simulink model "simulator"  (R2024a)
settings: Solver=VariableStepAuto  StartTime=0.0  StopTime=10  RelTol=1e-3
undefined symbols (not defined in the file): desiredState, params, x0
libraries: simulink x2, matrix_library x1
settings Model: Creator=matteocolussi  LastModifiedBy=matteocolussi

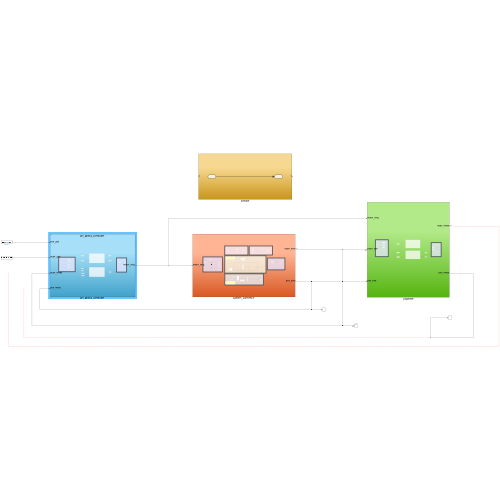
[thumbnail: Simulink's stored preview of the top-level diagram]
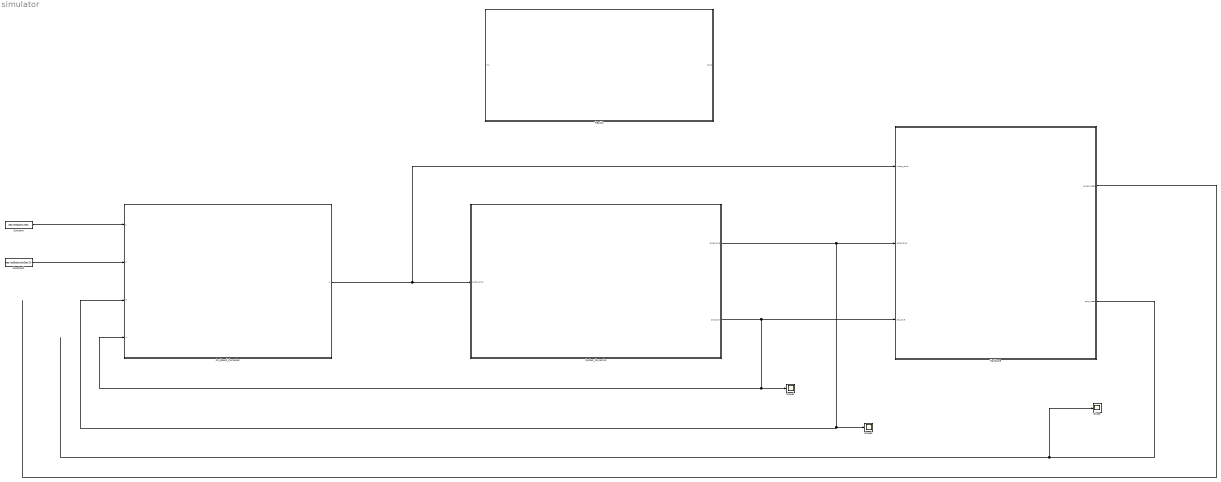
== system simulator ==
  Constant : Constant  Value=desiredState.rDes
  Constant1 : Constant  Value=desiredState.attDes(3)
  Hardware : Subsystem
  On_Board_Computer : Subsystem  ReferencedSubsystem=On_Board_Computer
  Results : Subsystem
  Scope : Scope
  Scope1 : Scope
  Scope2 : Scope
  System_Dynamics : Subsystem
  wires:
  On_Board_Computer/1 -> Hardware/1(motor_cmd), System_Dynamics/1(motor_cmd)
  System_Dynamics/1(euler_true) -> Hardware/2(euler_true), On_Board_Computer/3, Scope2/1
  System_Dynamics/2(pos_true) -> Scope1/1, On_Board_Computer/4, Hardware/3(pos_true)
  Hardware/1(euler_meas) -> ?
  Hardware/2(pos_meas) -> Scope/1
  Constant/1 -> On_Board_Computer/1
  Constant1/1 -> On_Board_Computer/2

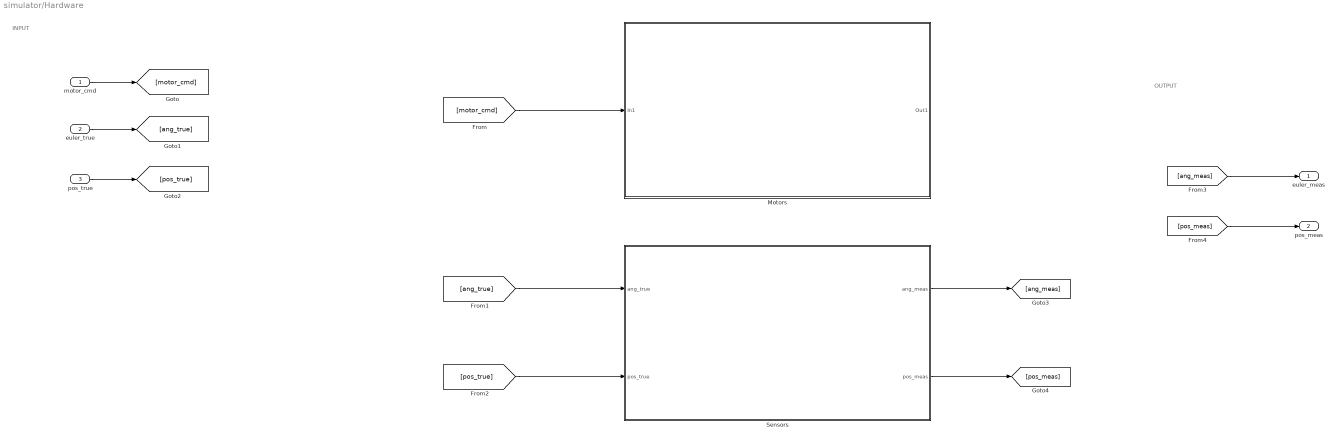
== system simulator/Hardware ==
  note: INPUT
  note: OUTPUT
  motor_cmd : Inport
  euler_true : Inport  Port=2
  pos_true : Inport  Port=3
  Motors : Subsystem
  Sensors : Subsystem
  euler_meas : Outport
  pos_meas : Outport  Port=2
  wires:
  motor_cmd/1 -> [motor_cmd]
  [motor_cmd] -> Motors/1(In1)
  euler_true/1 -> [ang_true]
  pos_true/1 -> [pos_true]
  [ang_true] -> Sensors/1(ang_true)
  [pos_true] -> Sensors/2(pos_true)
  Sensors/1(ang_meas) -> [ang_meas]
  Sensors/2(pos_meas) -> [pos_meas]
  [ang_meas] -> euler_meas/1
  [pos_meas] -> pos_meas/1

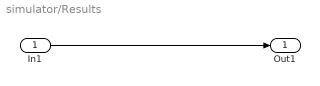
== system simulator/Results ==
  In1 : Inport
  Out1 : Outport
  wires:
  In1/1 -> Out1/1

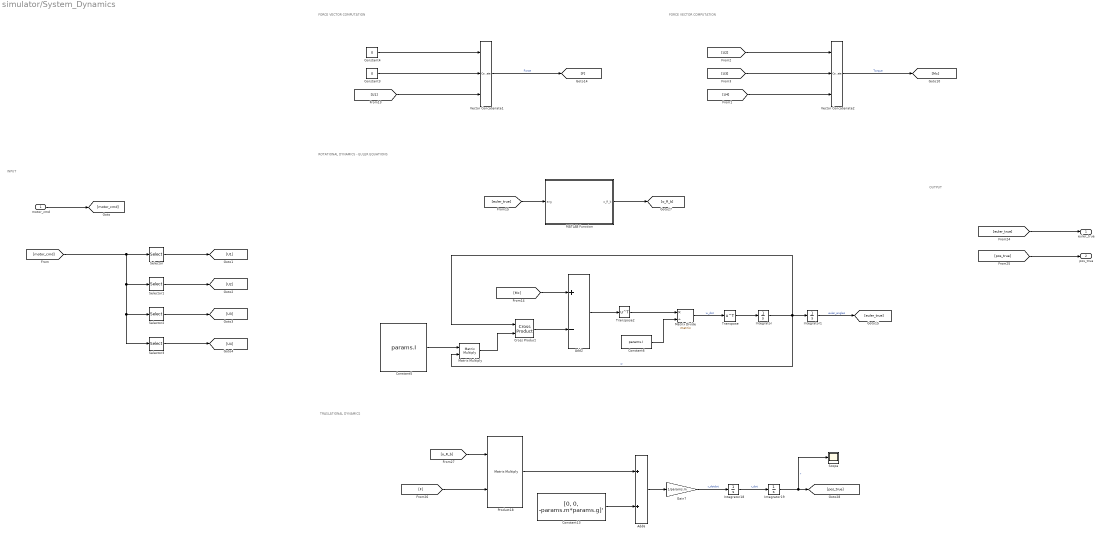
== system simulator/System_Dynamics ==
  note: ROTATIONAL DYNAMICS - EULER EQUATIONS
  note: FORCE VECTOR COMPUTATION
  note: INPUT
  note: OUTPUT
  note: TRASLATIONAL DYNAMICS
  note: FORCE VECTOR COMPUTATION
  motor_cmd : Inport
  Add2 : Sum  Inputs=+-
  Add6 : Sum
  Constant13 : Constant  Value=[0, 0, -params.m*params.g]'
  Constant3 : Constant  Value=0
  Constant4 : Constant  Value=0
  Constant5 : Constant  Value=params.I  VectorParams1D=off
  Constant6 : Constant  Value=params.I
  Cross Product : matrix_library/Cross Product
  Gain7 : Gain  Gain=1/params.m
  Integrator : Integrator
  Integrator1 : Integrator  InitialCondition=x0(7:9)
  Integrator18 : Integrator
  Integrator19 : Integrator  InitialCondition=x0(1:3);
  MATLAB Function : MATLAB Function  TreatAsAtomicUnit=on
  Matrix Divide : Product  Inputs=*/  Multiplication=Matrix(*)
  Matrix Multiply : Product  Multiplication=Matrix(*)
  Product18 : Product  Multiplication=Matrix(*)
  Scope : Scope
  Selector : Selector  InputPortWidth=4  IndexOptions=Index vector (dialog)  Indices=1  OutputSizes=1
  Selector1 : Selector  InputPortWidth=4  IndexOptions=Index vector (dialog)  Indices=2  OutputSizes=1
  Selector2 : Selector  InputPortWidth=4  IndexOptions=Index vector (dialog)  Indices=3  OutputSizes=1
  Selector3 : Selector  InputPortWidth=4  IndexOptions=Index vector (dialog)  Indices=4  OutputSizes=1
  Transpose : Math  Operator=transpose
  Transpose2 : Math  Operator=transpose
  Vector Concatenate1 : Concatenate  NumInputs=3
  Vector Concatenate2 : Concatenate  NumInputs=3
  euler_true : Outport
  pos_true : Outport  Port=2
  wires:
  motor_cmd/1 -> [motor_cmd]
  Selector/1 -> [U1]
  Selector1/1 -> [U2]
  Selector2/1 -> [U3]
  [motor_cmd] -> Selector3/1, Selector2/1, Selector1/1, Selector/1
  Selector3/1 -> [U4]
  [U1] -> Vector Concatenate1/3
  Constant3/1 -> Vector Concatenate1/2
  Constant4/1 -> Vector Concatenate1/1
  Vector Concatenate1/1 -> [F]  "Force"
  [euler_true] -> MATLAB Function/1(ang)
  MATLAB Function/1(o_R_b) -> [o_R_b]
  [euler_true] -> euler_true/1
  [pos_true] -> pos_true/1
  Add6/1 -> Gain7/1
  [F] -> Product18/2
  Product18/1 -> Add6/1
  Gain7/1 -> Integrator18/1  "r_dotdot"
  [o_R_b] -> Product18/1
  Constant13/1 -> Add6/2
  Integrator18/1 -> Integrator19/1  "r_dot"
  Integrator19/1 -> [pos_true], Scope/1  "r"
  Constant5/1 -> Matrix Multiply/1
  Matrix Multiply/1 -> Cross Product/2
  Cross Product/1 -> Add2/2
  Add2/1 -> Transpose2/1
  Constant6/1 -> Matrix Divide/2
  Matrix Divide/1 -> Transpose/1  "w_dot"
  Integrator/1 -> Integrator1/1, Cross Product/1, Matrix Multiply/2  "w"
  Integrator1/1 -> [euler_true]  "euler_angles"
  [U2] -> Vector Concatenate2/1
  Vector Concatenate2/1 -> [Mc]  "Torque"
  [U4] -> Vector Concatenate2/3
  [U3] -> Vector Concatenate2/2
  Transpose/1 -> Integrator/1
  [Mc] -> Add2/1
  Transpose2/1 -> Matrix Divide/1

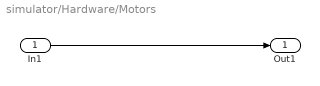
== system simulator/Hardware/Motors ==
  In1 : Inport
  Out1 : Outport
  wires:
  In1/1 -> Out1/1

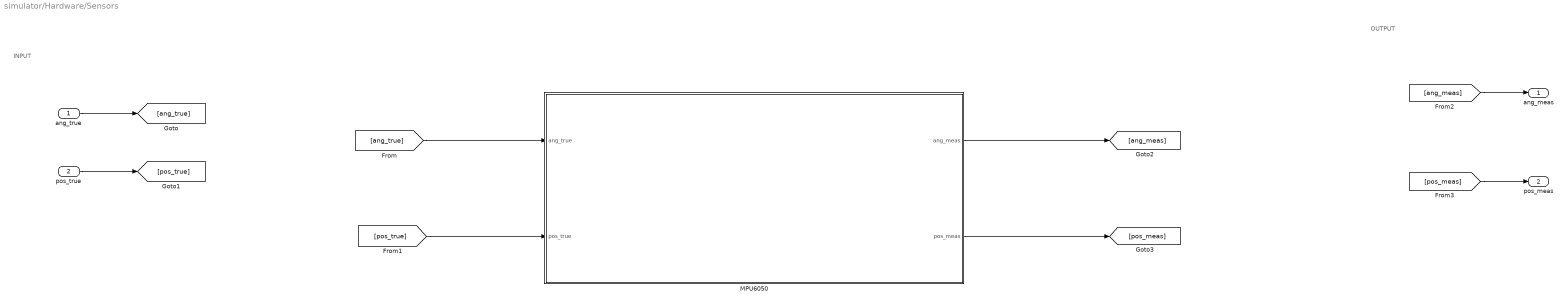
== system simulator/Hardware/Sensors ==
  note: OUTPUT
  note: INPUT
  ang_true : Inport
  pos_true : Inport  Port=2
  MPU6050 : Subsystem
  ang_meas : Outport
  pos_meas : Outport  Port=2
  wires:
  ang_true/1 -> [ang_true]
  pos_true/1 -> [pos_true]
  [ang_meas] -> ang_meas/1
  [pos_meas] -> pos_meas/1
  [ang_true] -> MPU6050/1(ang_true)
  [pos_true] -> MPU6050/2(pos_true)
  MPU6050/1(ang_meas) -> [ang_meas]
  MPU6050/2(pos_meas) -> [pos_meas]

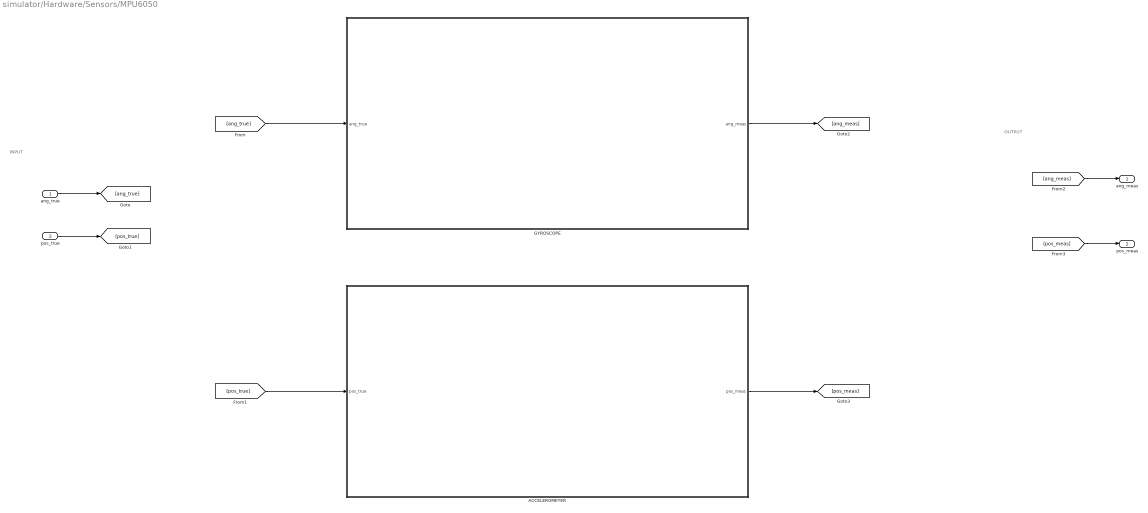
== system simulator/Hardware/Sensors/MPU6050 ==
  note: INPUT
  note: OUTPUT
  ang_true : Inport
  pos_true : Inport  Port=2
  ACCELEROMETER : Subsystem
  GYROSCOPE : Subsystem
  ang_meas : Outport
  pos_meas : Outport  Port=2
  wires:
  ang_true/1 -> [ang_true]
  pos_true/1 -> [pos_true]
  [pos_meas] -> pos_meas/1
  [ang_meas] -> ang_meas/1
  [ang_true] -> GYROSCOPE/1(ang_true)
  [pos_true] -> ACCELEROMETER/1(pos_true)
  GYROSCOPE/1(ang_meas) -> [ang_meas]
  ACCELEROMETER/1(pos_meas) -> [pos_meas]

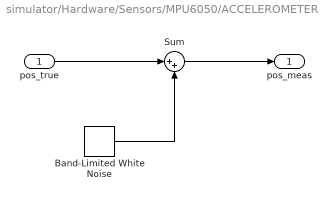
== system simulator/Hardware/Sensors/MPU6050/ACCELEROMETER ==
  pos_true : Inport
  Band-Limited White Noise : simulink/Sources/Band-Limited White Noise  Cov=[0.1]  Ts=0.1  seed=[23341]
  Sum : Sum  Inputs=|++
  pos_meas : Outport
  wires:
  Band-Limited White Noise/1 -> Sum/2
  pos_true/1 -> Sum/1
  Sum/1 -> pos_meas/1

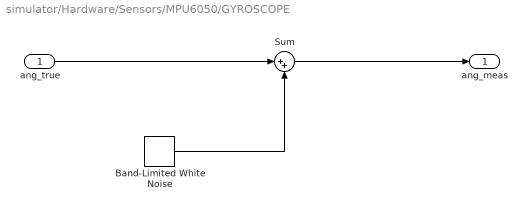
== system simulator/Hardware/Sensors/MPU6050/GYROSCOPE ==
  ang_true : Inport
  Band-Limited White Noise : simulink/Sources/Band-Limited White Noise  Cov=[0.1]  Ts=0.1  seed=[23341]
  Sum : Sum  Inputs=|++
  ang_meas : Outport
  wires:
  ang_true/1 -> Sum/1
  Band-Limited White Noise/1 -> Sum/2
  Sum/1 -> ang_meas/1

== matlab function simulator/System_Dynamics/MATLAB Function ==
  data: ang input; o_R_b output
function o_R_b  = RotMatrix(ang)

phi = ang(1);
theta = ang(2);
psi = ang(3);

o_R_b = zeros(3,3);

R_psi = [cos(psi),          -sin(psi),          0;
         sin(psi),           cos(psi),          0;
                0,                  0,          1];

R_theta = [cos(theta),              0,          sin(theta);
                    0,              1,                   0;
          -sin(theta),              0,          cos(theta)];

R_phi = [1,             0,              0;
         0,      cos(phi),      -sin(phi);
         0,      sin(phi),       cos(phi)];

o_R_b = R_psi * R_theta * R_phi;

end
